simulink model "Modelo5_1_2_C_6"  (R2020a)
settings: Solver=VariableStepAuto  StartTime=0.0  StopTime=50  MaxStep=1e-3  RelTol=1e-3
values from neighbouring files (symbols this model uses):
  aa = 3.9e-3    (= 0.0039)    [parametros.m]
  beq = bm+bl/(r^2)    (= 8.44444444444e-05)    [parametros.m]
  Cts = 0.818    [AnalisisDeEstabilidad.m]    (also in parametros.m)
  Jeq = Jm+Jl/(r^2)    (= 7.25444444444e-05)    [parametros.m]
  Kl = 1    [parametros.m]
  lam = 0.01546    [parametros.m]
  Ld = 5.8e-3    (= 0.0058)    [AnalisisDeEstabilidad.m]    (also in parametros.m = 0.0066)
  Lls = 0.8e-3    (= 0.0008)    [AnalisisDeEstabilidad.m]    (also in parametros.m)
  Lq = 6.6e-3    (= 0.0066)    [AnalisisDeEstabilidad.m]    (also in parametros.m = 0.0058)
  Pp = 3    [AnalisisDeEstabilidad.m]    (also in LTI_vs_LPV_vs_NL_realimentado.m; Modelo_linealizado.m; parametros.m)
  r = 120    [AnalisisDeEstabilidad.m]    (also in LTI_vs_LPV_vs_NL_realimentado.m; Modelo_linealizado.m; parametros.m)
  Rsref = 1.02    [AnalisisDeEstabilidad.m]    (also in parametros.m)
  Rts = 146.7    [AnalisisDeEstabilidad.m]    (also in parametros.m)
  Tref = 25    [AnalisisDeEstabilidad.m]    (also in parametros.m = 40)
libraries: simulink x2
settings Model: Creator=matie  LastModifiedBy=matie

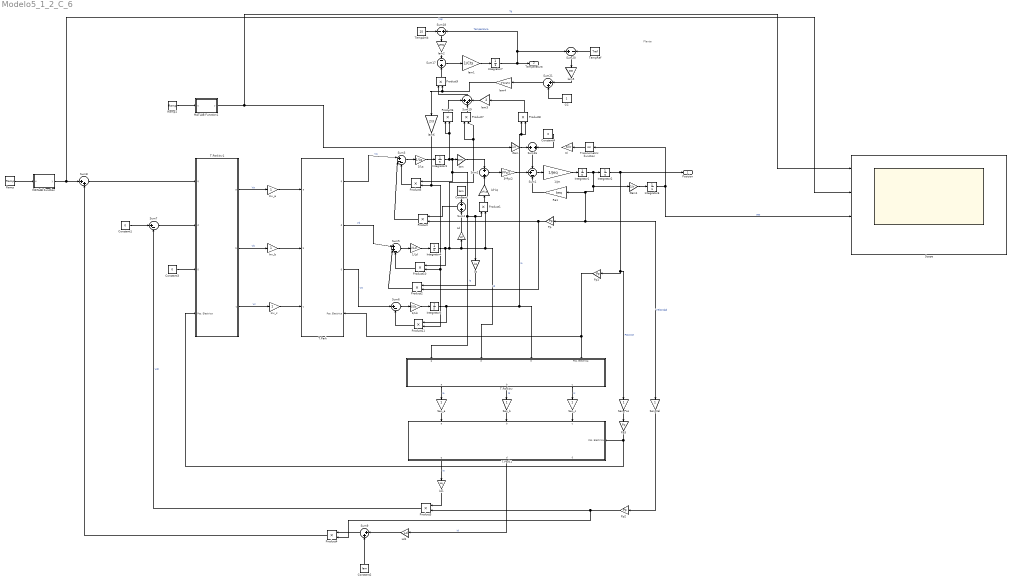
== system Modelo5_1_2_C_6 ==
  note: Planta
  1/Jm : Gain  Gain=1/Jeq
  1/Ld : Gain  Gain=1/Ld
  1/Lls : Gain  Gain=1/Lls
  1/Lq : Gain  Gain=1/Lq
  3*Pp/2 : Gain  Gain=3*Pp/2
  CC : Constant
  Constant : Constant  Value=lam
  Constant1 : Constant  Value=0
  Constant2 : Constant  Value=lam
  Constant3 : Constant  Value=0
  Constant4 : Constant  Value=0
  Gain : Gain  Gain=1/r
  Gain1 : Gain  Gain=1/r
  Integrator{1..7} (7 alike) : Integrator
  Inv_a : Gain
  Inv_b : Gain
  Inv_c : Gain
  Kl : Gain  Gain=Kl/r
  Ld : Gain  Gain=Ld
  Ld-Lq : Gain  Gain=Ld-Lq
  Ld1 : Gain  Gain=Ld
  Lq : Gain  Gain=Lq
  Lq1 : Gain  Gain=Lq
  MATLAB Function : MATLAB Function  TreatAsAtomicUnit=on
  MATLAB Function1 : MATLAB Function  TreatAsAtomicUnit=on
  Pp{,1..3} (4 alike) : Gain  Gain=Pp
  Product{,1..11} (12 alike) : Product
  Ra1 : Gain  Gain=beq
  Ramp : simulink/Sources/Ramp  slope=0  start=0  InitialOutput=0
  Ramp1 : simulink/Sources/Ramp  slope=1  start=0  InitialOutput=0
  Scope : Scope  NumInputPorts=4
  Sen_Pos : Gain
  Sen_Vel : Gain
  Sen_a : Gain
  Sen_b : Gain
  Sen_c : Gain
  Sum1 : Sum  Inputs=-+-
  Sum16 : Sum  Inputs=+|+
  Sum17 : Sum  Inputs=-+
  Sum18 : Sum  Inputs=-+
  Sum19 : Sum  Inputs=+++
  Sum2 : Sum
  Sum20 : Sum  Inputs=+-
  Sum21 : Sum  Inputs=|++
  Sum3 : Sum  Inputs=|+--
  Sum4 : Sum
  Sum5 : Sum  Inputs=|++-
  Sum6 : Sum  Inputs=|+-
  Sum7 : Sum  Inputs=|+-
  Sum8 : Sum  Inputs=|++
  Sum9 : Sum  Inputs=|++
  T.Park : Subsystem
      settings: PortSchema="{\"entries\":[{\"content\":{\"sides\":[{\"content\":{\"connectorIds\":[\"In1\",\"In2\",\"In3\"]},\"type\":\"ConnectorPlacement.EquallySpacedRectSide\",\"uuid\":\"2bfbe7ef-652a-4797-b13c-b84c243bd68c\"},{\"content\":{\"connectorIds\":[\"Out1\",\"Out2\",\"Out3\",\"In4\"],\"side\":\"RIGHT\"},\"type\":\"ConnectorPlacement.EquallySpacedRectSide\",\"uuid\":\"075def0e-c436-44dc-ba25-82cf6ffae869\"},{\"content\":{\"connectorIds\":[],\"side\":\"TOP\"},\"type\":\"ConnectorPlacement.EquallySpacedRectSide\",\"uuid\":\"95d81334-e332-4f04-a2cb-c4692f91809c\"}]},\"type\":\"ConnectorPlacement.EquallySpacedConnector\",\"uuid\":\"b90f9cad-0277-459c-bcac-17172872a787\"}],\"packageUris\":[\"http://schema.mathworks.com/mf0/Connector/19700101\"],\"version\":\"1.0\"}"
  T.Park1 : Subsystem
      settings: PortSchema="{\"entries\":[{\"content\":{\"sides\":[{\"content\":{\"connectorIds\":[\"In1\",\"In2\",\"In3\"]},\"type\":\"ConnectorPlacement.EquallySpacedRectSide\",\"uuid\":\"2bfbe7ef-652a-4797-b13c-b84c243bd68c\"},{\"content\":{\"connectorIds\":[\"Out1\",\"Out2\",\"Out3\"],\"side\":\"RIGHT\"},\"type\":\"ConnectorPlacement.EquallySpacedRectSide\",\"uuid\":\"075def0e-c436-44dc-ba25-82cf6ffae869\"},{\"content\":{\"connectorIds\":[],\"side\":\"TOP\"},\"type\":\"ConnectorPlacement.EquallySpacedRectSide\",\"uuid\":\"95d81334-e332-4f04-a2cb-c4692f91809c\"},{\"content\":{\"connectorIds\":[\"In4\"],\"side\":\"BOTTOM\"},\"type\":\"ConnectorPlacement.EquallySpacedRectSide\",\"uuid\":\"85b95360-e43d-49d1-a18f-690334b045e6\"}]},\"type\":\"ConnectorPlacement.EquallySpacedConnector\",\"uuid\":\"b90f9cad-0277-459c-bcac-17172872a787\"}],\"packageUris\":[\"http://schema.mathworks.com/mf0/Connector/19700101\"],\"version\":\"1.0\"}"
  T.ParkInv : Subsystem
  T.ParkInv1 : Subsystem
  TempAmb : Constant  Value=25
  TempRef : Constant  Value=Tref
  Trigonometric Function : Trigonometry
  lam : Gain  Gain=lam
  lam1 : Gain  Gain=1/Cts
  lam2 : Gain  Gain=1/Rts
  lam3 : Gain  Gain=2
  lam4 : Gain  Gain=3*Rsref/2
  lam5 : Gain  Gain=aa
  lam6 : Gain  Gain=2/3
  Posicion : Outport
  Temperatura : Outport  Port=2
  wires:
  Integrator6/1 -> Trigonometric Function/1, Scope/3  "pos"
  Inv_b/1 -> T.Park/2(b)
  Pp3/1 -> T.ParkInv1/4(Pos. Electrica), T.Park1/4(Pos. Electrica)
  Sum1/1 -> 1/Jm/1
  Sum17/1 -> lam1/1
  Integrator5/1 -> Product11/1, T.ParkInv/3(0), Product8/2, Product8/1  "io"
  Sum19/1 -> Product9/1
  1/Jm/1 -> Integrator1/1
  Lq1/1 -> Product3/1
  lam4/1 -> lam6/1, Product9/2
  Integrator3/1 -> Product6/1, Product6/2, Product5/1, Product1/1, Lq/1, T.ParkInv/1(q), lam/1  "iq"
  Integrator7/1 -> Sum18/2, Sum20/1, Temperatura/1  "Temperatura"
  T.ParkInv/1(a) -> Sen_a/1  "Ia"
  Pp2/1 -> Product4/2, Product3/2
  Pp/1 -> Product2/2, Product/2
  Product5/1 -> Sum3/3
  Sum21/1 -> lam4/1
  Product7/1 -> Sum19/2
  Integrator1/1 -> Gain1/1, Sen_Vel/1, Pp/1, Ra1/1, Integrator2/1  "Velocidad"
  TempRef/1 -> Sum20/2
  Product3/1 -> Sum7/2  "Vd*"
  Product2/1 -> Sum5/2
  Sum3/1 -> 1/Lq/1
  Pp1/1 -> T.Park/4(Pos. Electrica), T.ParkInv/4(Pos. Electrica)
  T.Park1/1(q) -> Lq1/1  "iq"
  Lq/1 -> Product2/1
  Product6/1 -> Sum19/1
  Integrator2/1 -> Sen_Pos/1, Pp1/1, Posicion/1  "Posicion"
  T.ParkInv/3(c) -> Sen_c/1  "Ic"
  T.Park/2(d) -> Sum5/1  "Vd"
  Product11/1 -> Sum6/2
  Sum6/1 -> 1/Lls/1
  1/Lls/1 -> Integrator5/1
  Sum4/1 -> Product/1
  CC/1 -> Sum21/2
  Inv_a/1 -> T.Park/1(a)
  T.ParkInv1/3(c) -> Inv_c/1  "Vc"
  T.Park/3(0) -> Sum6/1  "V0"
  Sum5/1 -> 1/Ld/1
  lam/1 -> Sum2/1
  T.Park/1(q) -> Sum3/1  "Vq"
  Integrator4/1 -> Product10/1, Product7/1, Product7/2, Product1/2, T.ParkInv/2(d), Ld/1  "id"
  Gain1/1 -> Integrator6/1
  lam1/1 -> Integrator7/1
  Sum18/1 -> lam2/1
  Ra1/1 -> Sum1/3
  MATLAB Function1/1(y) -> Scope/1, Gain/1  "Td"
  T.ParkInv/2(b) -> Sen_b/1  "Ib"
  TempAmb/1 -> Sum18/1
  Ld-Lq/1 -> Sum2/2
  T.ParkInv1/2(b) -> Inv_b/1  "Vb"
  Sen_c/1 -> T.Park1/3(c)
  Sum20/1 -> lam5/1
  Trigonometric Function/1 -> Kl/1
  Sen_b/1 -> T.Park1/2(b)
  Product8/1 -> lam3/1
  3*Pp/2/1 -> Sum1/2
  Sen_a/1 -> T.Park1/1(a)
  Product10/1 -> Sum5/3
  lam3/1 -> Sum19/3
  Product1/1 -> Ld-Lq/1
  Product9/1 -> Sum17/2
  Constant/1 -> Sum4/1
  Sum16/1 -> Sum1/1
  lam5/1 -> Sum21/1
  Ld/1 -> Sum4/2
  Inv_c/1 -> T.Park/3(c)
  lam2/1 -> Sum17/1
  Sum2/1 -> 3*Pp/2/1
  1/Ld/1 -> Integrator4/1
  T.ParkInv1/1(a) -> Inv_a/1  "Va"
  Sen_Pos/1 -> Pp3/1
  Gain/1 -> Sum16/1
  Product/1 -> Sum3/2
  1/Lq/1 -> Integrator3/1
  Sum7/1 -> T.ParkInv1/2(d)
  Constant1/1 -> Sum7/1
  Constant2/1 -> Sum9/2
  Ld1/1 -> Sum9/1
  Sum9/1 -> Product4/1
  T.Park1/2(d) -> Ld1/1  "id"
  Product4/1 -> Sum8/2
  Sen_Vel/1 -> Pp2/1
  Sum8/1 -> T.ParkInv1/1(q)
  MATLAB Function/1(y) -> Scope/2, Sum8/1  "Vqs"
  Ramp/1 -> MATLAB Function/1(u)
  Ramp1/1 -> MATLAB Function1/1(u)
  Constant3/1 -> T.ParkInv1/3(0)
  lam6/1 -> Product5/2, Product11/2, Product10/2
  Constant4/1 -> Sum16/2

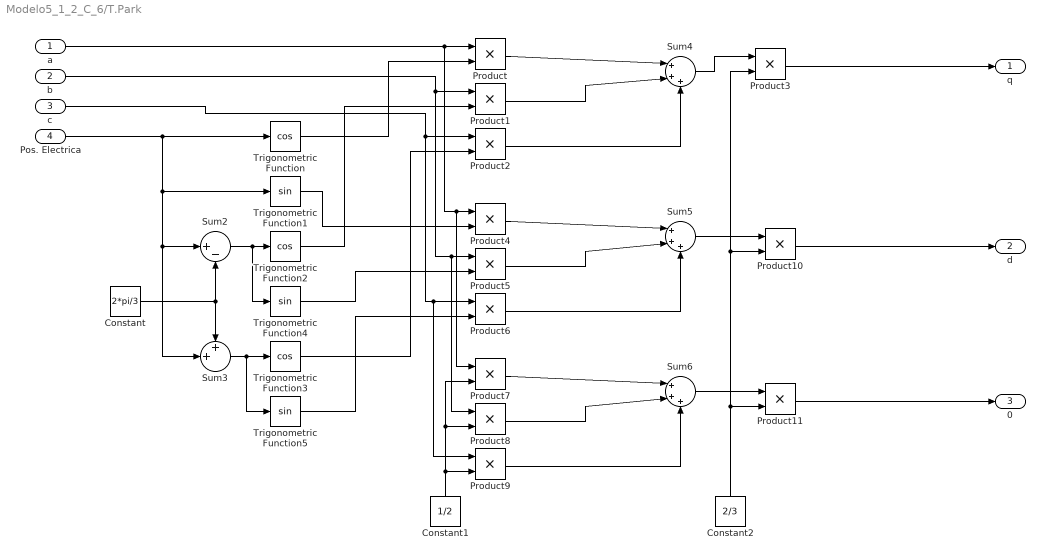
== system Modelo5_1_2_C_6/T.Park ==
  a : Inport
  b : Inport  Port=2
  c : Inport  Port=3
  Pos. Electrica : Inport  Port=4
  Constant : Constant  Value=2*pi/3
  Constant1 : Constant  Value=1/2
  Constant2 : Constant  Value=2/3
  Product{,1..11} (12 alike) : Product
  Sum2 : Sum  Inputs=|+-
  Sum3 : Sum  Inputs=++|
  Sum4 : Sum  Inputs=|+++
  Sum5 : Sum  Inputs=|+++
  Sum6 : Sum  Inputs=|+++
  Trigonometric Function : Trigonometry  Operator=cos
  Trigonometric Function1 : Trigonometry
  Trigonometric Function2 : Trigonometry  Operator=cos
  Trigonometric Function3 : Trigonometry  Operator=cos
  Trigonometric Function4 : Trigonometry
  Trigonometric Function5 : Trigonometry
  q : Outport
  d : Outport  Port=2
  0 : Outport  Port=3
  wires:
  Product1/1 -> Sum4/2
  c/1 -> Product9/1, Product6/1, Product2/1
  Constant1/1 -> Product9/2, Product8/2, Product7/2
  Sum2/1 -> Trigonometric Function4/1, Trigonometric Function2/1
  Constant2/1 -> Product11/2, Product10/2, Product3/2
  b/1 -> Product8/1, Product5/1, Product1/1
  Product11/1 -> 0/1
  Pos. Electrica/1 -> Sum3/2, Sum2/1, Trigonometric Function1/1, Trigonometric Function/1
  Trigonometric Function2/1 -> Product1/2
  Trigonometric Function5/1 -> Product6/2
  Product6/1 -> Sum5/3
  Trigonometric Function1/1 -> Product4/2
  Constant/1 -> Sum3/1, Sum2/2
  Sum5/1 -> Product10/1
  Product3/1 -> q/1
  Sum4/1 -> Product3/1
  Trigonometric Function3/1 -> Product2/2
  Trigonometric Function/1 -> Product/2
  a/1 -> Product7/1, Product4/1, Product/1
  Product10/1 -> d/1
  Trigonometric Function4/1 -> Product5/2
  Product/1 -> Sum4/1
  Product7/1 -> Sum6/1
  Sum3/1 -> Trigonometric Function5/1, Trigonometric Function3/1
  Product2/1 -> Sum4/3
  Product9/1 -> Sum6/3
  Product5/1 -> Sum5/2
  Product4/1 -> Sum5/1
  Sum6/1 -> Product11/1
  Product8/1 -> Sum6/2

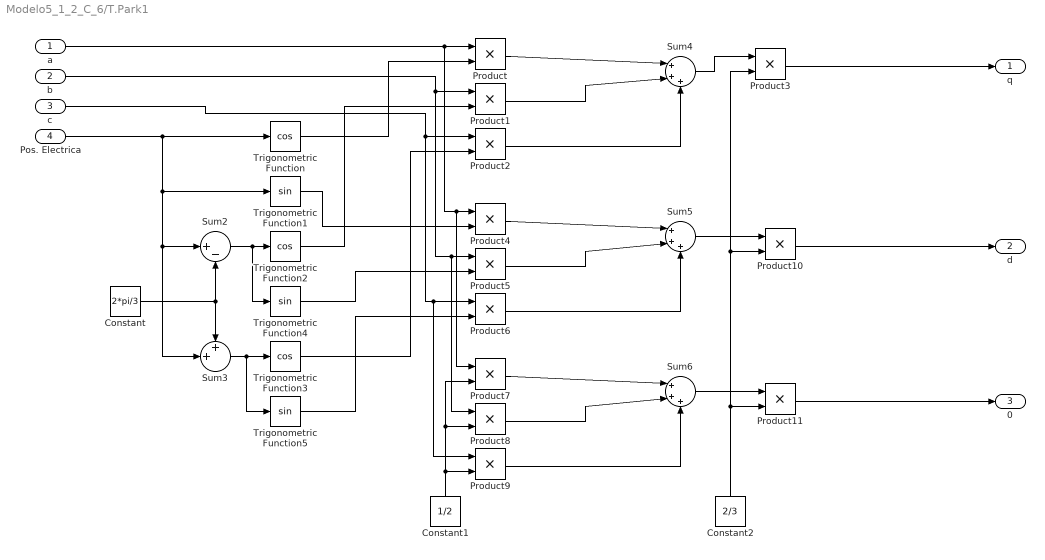
== system Modelo5_1_2_C_6/T.Park1 ==
  a : Inport
  b : Inport  Port=2
  c : Inport  Port=3
  Pos. Electrica : Inport  Port=4
  Constant : Constant  Value=2*pi/3
  Constant1 : Constant  Value=1/2
  Constant2 : Constant  Value=2/3
  Product{,1..11} (12 alike) : Product
  Sum2 : Sum  Inputs=|+-
  Sum3 : Sum  Inputs=++|
  Sum4 : Sum  Inputs=|+++
  Sum5 : Sum  Inputs=|+++
  Sum6 : Sum  Inputs=|+++
  Trigonometric Function : Trigonometry  Operator=cos
  Trigonometric Function1 : Trigonometry
  Trigonometric Function2 : Trigonometry  Operator=cos
  Trigonometric Function3 : Trigonometry  Operator=cos
  Trigonometric Function4 : Trigonometry
  Trigonometric Function5 : Trigonometry
  q : Outport
  d : Outport  Port=2
  0 : Outport  Port=3
  wires:
  Product1/1 -> Sum4/2
  c/1 -> Product9/1, Product6/1, Product2/1
  Constant1/1 -> Product9/2, Product8/2, Product7/2
  Sum2/1 -> Trigonometric Function4/1, Trigonometric Function2/1
  Constant2/1 -> Product11/2, Product10/2, Product3/2
  b/1 -> Product8/1, Product5/1, Product1/1
  Product11/1 -> 0/1
  Pos. Electrica/1 -> Sum3/2, Sum2/1, Trigonometric Function1/1, Trigonometric Function/1
  Trigonometric Function2/1 -> Product1/2
  Trigonometric Function5/1 -> Product6/2
  Product6/1 -> Sum5/3
  Trigonometric Function1/1 -> Product4/2
  Constant/1 -> Sum3/1, Sum2/2
  Sum5/1 -> Product10/1
  Product3/1 -> q/1
  Sum4/1 -> Product3/1
  Trigonometric Function3/1 -> Product2/2
  Trigonometric Function/1 -> Product/2
  a/1 -> Product7/1, Product4/1, Product/1
  Product10/1 -> d/1
  Trigonometric Function4/1 -> Product5/2
  Product/1 -> Sum4/1
  Product7/1 -> Sum6/1
  Sum3/1 -> Trigonometric Function5/1, Trigonometric Function3/1
  Product2/1 -> Sum4/3
  Product9/1 -> Sum6/3
  Product5/1 -> Sum5/2
  Product4/1 -> Sum5/1
  Sum6/1 -> Product11/1
  Product8/1 -> Sum6/2

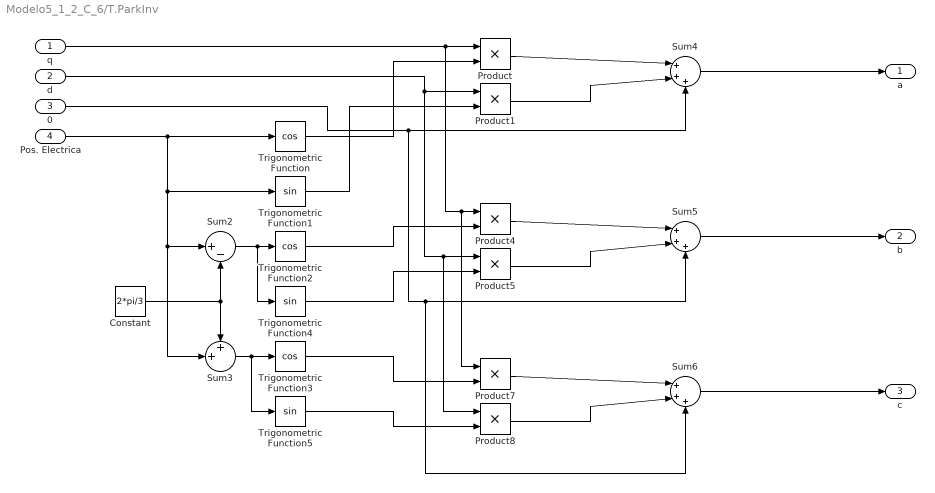
== system Modelo5_1_2_C_6/T.ParkInv ==
  q : Inport
  d : Inport  Port=2
  0 : Inport  Port=3
  Pos. Electrica : Inport  Port=4
  Constant : Constant  Value=2*pi/3
  Product{,1,4..5,7..8} (6 alike) : Product
  Sum2 : Sum  Inputs=|+-
  Sum3 : Sum  Inputs=++|
  Sum4 : Sum  Inputs=|+++
  Sum5 : Sum  Inputs=|+++
  Sum6 : Sum  Inputs=|+++
  Trigonometric Function : Trigonometry  Operator=cos
  Trigonometric Function1 : Trigonometry
  Trigonometric Function2 : Trigonometry  Operator=cos
  Trigonometric Function3 : Trigonometry  Operator=cos
  Trigonometric Function4 : Trigonometry
  Trigonometric Function5 : Trigonometry
  a : Outport
  b : Outport  Port=2
  c : Outport  Port=3
  wires:
  Constant/1 -> Sum3/1, Sum2/2
  Pos. Electrica/1 -> Sum3/2, Sum2/1, Trigonometric Function1/1, Trigonometric Function/1
  Trigonometric Function3/1 -> Product7/2
  d/1 -> Product8/1, Product5/1, Product1/1
  0/1 -> Sum4/3, Sum5/3, Sum6/3
  Product8/1 -> Sum6/2
  Product7/1 -> Sum6/1
  q/1 -> Product7/1, Product4/1, Product/1
  Sum3/1 -> Trigonometric Function5/1, Trigonometric Function3/1
  Trigonometric Function5/1 -> Product8/2
  Sum6/1 -> c/1
  Product1/1 -> Sum4/2
  Sum2/1 -> Trigonometric Function4/1, Trigonometric Function2/1
  Sum4/1 -> a/1
  Sum5/1 -> b/1
  Trigonometric Function1/1 -> Product1/2
  Product5/1 -> Sum5/2
  Trigonometric Function2/1 -> Product4/2
  Product4/1 -> Sum5/1
  Product/1 -> Sum4/1
  Trigonometric Function/1 -> Product/2
  Trigonometric Function4/1 -> Product5/2

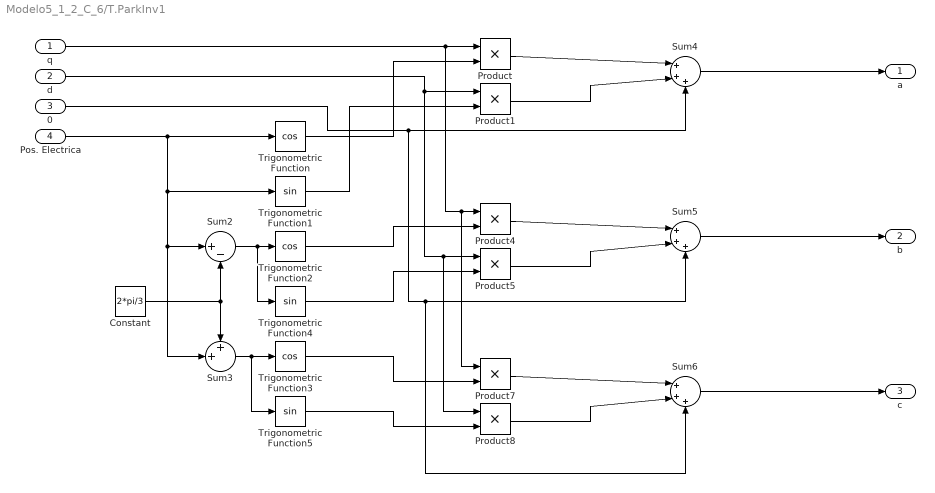
== system Modelo5_1_2_C_6/T.ParkInv1 ==
  q : Inport
  d : Inport  Port=2
  0 : Inport  Port=3
  Pos. Electrica : Inport  Port=4
  Constant : Constant  Value=2*pi/3
  Product{,1,4..5,7..8} (6 alike) : Product
  Sum2 : Sum  Inputs=|+-
  Sum3 : Sum  Inputs=++|
  Sum4 : Sum  Inputs=|+++
  Sum5 : Sum  Inputs=|+++
  Sum6 : Sum  Inputs=|+++
  Trigonometric Function : Trigonometry  Operator=cos
  Trigonometric Function1 : Trigonometry
  Trigonometric Function2 : Trigonometry  Operator=cos
  Trigonometric Function3 : Trigonometry  Operator=cos
  Trigonometric Function4 : Trigonometry
  Trigonometric Function5 : Trigonometry
  a : Outport
  b : Outport  Port=2
  c : Outport  Port=3
  wires:
  Constant/1 -> Sum3/1, Sum2/2
  Pos. Electrica/1 -> Sum3/2, Sum2/1, Trigonometric Function1/1, Trigonometric Function/1
  Trigonometric Function3/1 -> Product7/2
  d/1 -> Product8/1, Product5/1, Product1/1
  0/1 -> Sum4/3, Sum5/3, Sum6/3
  Product8/1 -> Sum6/2
  Product7/1 -> Sum6/1
  q/1 -> Product7/1, Product4/1, Product/1
  Sum3/1 -> Trigonometric Function5/1, Trigonometric Function3/1
  Trigonometric Function5/1 -> Product8/2
  Sum6/1 -> c/1
  Product1/1 -> Sum4/2
  Sum2/1 -> Trigonometric Function4/1, Trigonometric Function2/1
  Sum4/1 -> a/1
  Sum5/1 -> b/1
  Trigonometric Function1/1 -> Product1/2
  Product5/1 -> Sum5/2
  Trigonometric Function2/1 -> Product4/2
  Product4/1 -> Sum5/1
  Product/1 -> Sum4/1
  Trigonometric Function/1 -> Product/2
  Trigonometric Function4/1 -> Product5/2

== matlab function Modelo5_1_2_C_6/MATLAB Function ==
  data: u input; y output
function y = fcn(u)
y = 0;
if (u>=0.1)&&(u<=0.7)
    y = 19.596;
end

== matlab function Modelo5_1_2_C_6/MATLAB Function1 ==
  data: u input; y output
function y = fcn(u)
y = 0;
if (u>=0.3)&&(u<=0.5)
    y = 6.28;
end
if (u>0.5)&&(u<=0.9)
    y = -6.28;
end
